simulink model "MultiMobileRobotObstacleAvoidance"  (R2020b)
settings: Solver=VariableStepAuto  StartTime=0.0  StopTime=100  RelTol=1e-3
values from neighbouring files (symbols this model uses):
  initTheta1 = -pi/2    (= -1.57079632679)    [createEnvMulti.m]
  initTheta2 = -pi/2    (= -1.57079632679)    [createEnvMulti.m]
  initX1 = 5    [createEnvMulti.m]
  initX2 = 22    [createEnvMulti.m]
  initY1 = 22    [createEnvMulti.m]
  initY2 = 22    [createEnvMulti.m]
  lidarNoiseSeeds = randi(intmax,size(scanAngles))    [createEnvMulti.m]
  lidarNoiseVariance = 0.1^2    (= 0.01)    [createEnvMulti.m]
  mapMatrix = simpleMap    [createEnvMulti.m]
  maxAngSpeed = 0.3    [createEnvMulti.m]
  maxLinSpeed = 0.3    [createEnvMulti.m]
  maxRange = 12    [createEnvMulti.m]
  sampleTime = 0.1    [createEnvMulti.m]
libraries: simulink x6, rllib x2, robotmobilelib x2
settings Model: Creator=fan  LastModifiedBy=fanyang

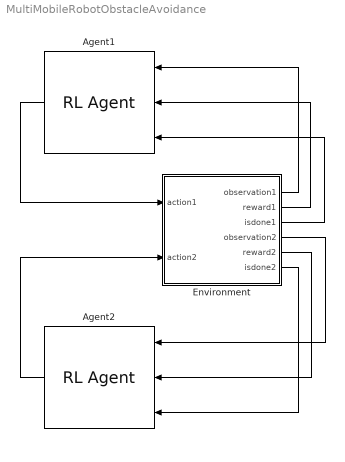
== system MultiMobileRobotObstacleAvoidance ==
  Agent1 : rllib/RL Agent  Agent=obstacleAvoidanceAgent1  ProvideReward=on  ProvideIsDone=on  ProvideCumRwd=off  TreatAsDirectFeedthrough=on  CollectLoggedSignals=on  CollectModelStates=on
  Agent2 : rllib/RL Agent  Agent=obstacleAvoidanceAgent2  ProvideReward=on  ProvideIsDone=on  ProvideCumRwd=off  TreatAsDirectFeedthrough=on  CollectLoggedSignals=on  CollectModelStates=on
  Environment : Subsystem
  wires:
  Environment/6(isdone2) -> Agent2/3
  Agent2/1 -> Environment/2(action2)
  Environment/3(isdone1) -> Agent1/3
  Environment/4(observation2) -> Agent2/1
  Environment/5(reward2) -> Agent2/2
  Environment/1(observation1) -> Agent1/1
  Environment/2(reward1) -> Agent1/2
  Agent1/1 -> Environment/1(action1)

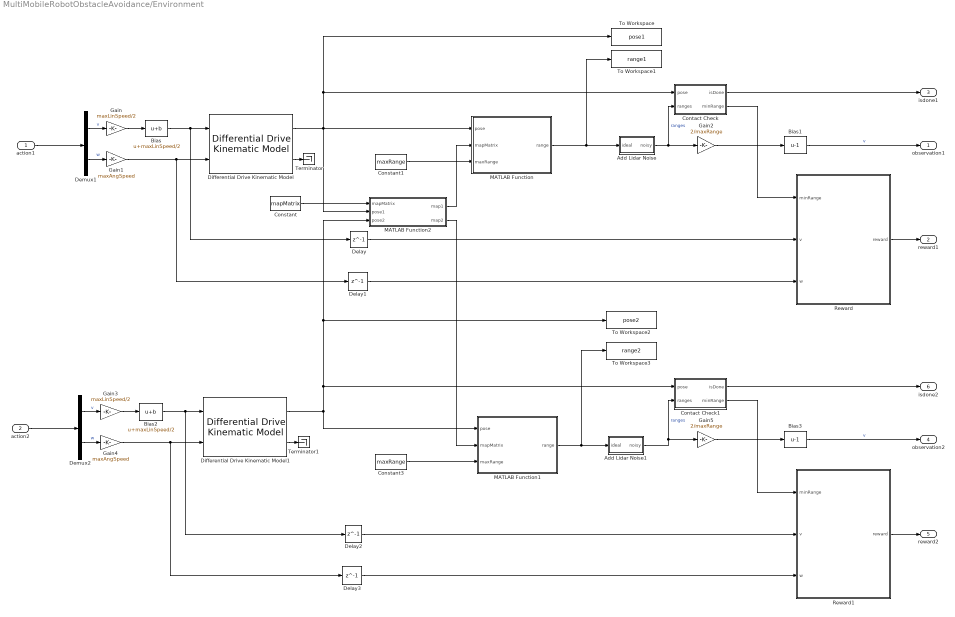
== system MultiMobileRobotObstacleAvoidance/Environment ==
  action1 : Inport
  action2 : Inport  Port=2
  Add Lidar Noise : Subsystem
  Add Lidar Noise1 : Subsystem
  Bias : Bias  Bias=maxLinSpeed/2
  Bias1 : Bias  Bias=-1
  Bias2 : Bias  Bias=maxLinSpeed/2
  Bias3 : Bias  Bias=-1
  Constant : Constant  Value=mapMatrix
  Constant1 : Constant  Value=maxRange
  Constant3 : Constant  Value=maxRange
  Contact Check : Subsystem
  Contact Check1 : Subsystem
  Delay{,1..3} (4 alike) : Delay  DelayLength=1  InitialCondition=0  UseCircularBuffer=on
  Demux1 : Demux  Outputs=2
  Demux2 : Demux  Outputs=2
  Differential Drive Kinematic Model : robotmobilelib/Differential Drive Kinematic Model  VehicleInputs=Vehicle Speed & Heading Angular Velocity  WheelRadius=0.05  WheelSpeedRange=[-inf inf]  TrackWidth=0.2  InitialState=[initX1; initY1; initTheta1]  SimulateUsing=Code generation
      settings: SourceProductBaseCode=RO
  Differential Drive Kinematic Model1 : robotmobilelib/Differential Drive Kinematic Model  VehicleInputs=Vehicle Speed & Heading Angular Velocity  WheelRadius=0.05  WheelSpeedRange=[-inf inf]  TrackWidth=0.2  InitialState=[initX2; initY2; initTheta2]  SimulateUsing=Code generation
      settings: SourceProductBaseCode=RO
  Gain : Gain  Gain=maxLinSpeed/2
  Gain1 : Gain  Gain=maxAngSpeed
  Gain2 : Gain  Gain=2/maxRange
  Gain3 : Gain  Gain=maxLinSpeed/2
  Gain4 : Gain  Gain=maxAngSpeed
  Gain5 : Gain  Gain=2/maxRange
  MATLAB Function : MATLAB Function  TreatAsAtomicUnit=on
  MATLAB Function1 : MATLAB Function  TreatAsAtomicUnit=on
  MATLAB Function2 : MATLAB Function  TreatAsAtomicUnit=on
  Reward : Subsystem
  Reward1 : Subsystem
  Terminator : Terminator
  Terminator1 : Terminator
  To Workspace : ToWorkspace  VariableName=pose1  SampleTime=-1
      settings: Save2DSignal=2-D array (concatenate along first dimension)
  To Workspace1 : ToWorkspace  VariableName=range1  SampleTime=-1
  To Workspace2 : ToWorkspace  VariableName=pose2  SampleTime=-1
      settings: Save2DSignal=2-D array (concatenate along first dimension)
  To Workspace3 : ToWorkspace  VariableName=range2  SampleTime=-1
  observation1 : Outport
  reward1 : Outport  Port=2
  isdone1 : Outport  Port=3
  observation2 : Outport  Port=4
  reward2 : Outport  Port=5
  isdone2 : Outport  Port=6
  wires:
  Differential Drive Kinematic Model/2 -> Terminator/1
  Differential Drive Kinematic Model/1 -> To Workspace/1, Contact Check/1(pose), MATLAB Function2/2(pose1), MATLAB Function/1(pose)
  action1/1 -> Demux1/1
  Bias/1 -> Delay/1, Differential Drive Kinematic Model/1
  Gain1/1 -> Delay1/1, Differential Drive Kinematic Model/2
  MATLAB Function/1(range) -> Add Lidar Noise/1(ideal), To Workspace1/1
  Contact Check/1(isDone) -> isdone1/1
  Contact Check/2(minRange) -> Reward/1(minRange)
  Reward/1(reward) -> reward1/1
  Gain2/1 -> Bias1/1
  Bias1/1 -> observation1/1  "v"
  Constant1/1 -> MATLAB Function/3(maxRange)
  Delay/1 -> Reward/2(v)
  Delay1/1 -> Reward/3(w)
  Demux1/2 -> Gain1/1  "w"
  Gain/1 -> Bias/1
  Demux1/1 -> Gain/1  "v"
  Add Lidar Noise/1(noisy) -> Gain2/1, Contact Check/2(ranges)  "ranges"
  Constant3/1 -> MATLAB Function1/3(maxRange)
  Delay2/1 -> Reward1/2(v)
  Add Lidar Noise1/1(noisy) -> Gain5/1, Contact Check1/2(ranges)  "ranges"
  Bias2/1 -> Delay2/1, Differential Drive Kinematic Model1/1
  Delay3/1 -> Reward1/3(w)
  Demux2/1 -> Gain3/1  "v"
  Demux2/2 -> Gain4/1  "w"
  Differential Drive Kinematic Model1/2 -> Terminator1/1
  Gain5/1 -> Bias3/1
  Gain3/1 -> Bias2/1
  action2/1 -> Demux2/1
  Reward1/1(reward) -> reward2/1
  Gain4/1 -> Delay3/1, Differential Drive Kinematic Model1/2
  Bias3/1 -> observation2/1  "v"
  Contact Check1/1(isDone) -> isdone2/1
  Contact Check1/2(minRange) -> Reward1/1(minRange)
  MATLAB Function1/1(range) -> To Workspace3/1, Add Lidar Noise1/1(ideal)
  Differential Drive Kinematic Model1/1 -> MATLAB Function2/3(pose2), To Workspace2/1, Contact Check1/1(pose), MATLAB Function1/1(pose)
  Constant/1 -> MATLAB Function2/1(mapMatrix)
  MATLAB Function2/1(map1) -> MATLAB Function/2(mapMatrix)
  MATLAB Function2/2(map2) -> MATLAB Function1/2(mapMatrix)

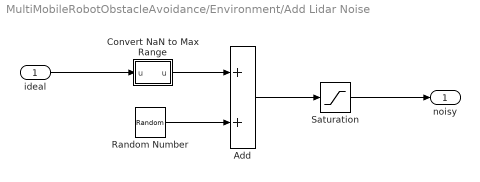
== system MultiMobileRobotObstacleAvoidance/Environment/Add Lidar Noise ==
  ideal : Inport
  Add : Sum
  Convert NaN to Max Range : MATLAB Function  TreatAsAtomicUnit=on
  Random Number : RandomNumber  Variance=lidarNoiseVariance  Seed=lidarNoiseSeeds  SampleTime=sampleTime
  Saturation : Saturate  UpperLimit=inf  LowerLimit=0
  noisy : Outport
  wires:
  Random Number/1 -> Add/2
  Add/1 -> Saturation/1
  Saturation/1 -> noisy/1
  ideal/1 -> Convert NaN to Max Range/1("u ")
  Convert NaN to Max Range/1(u) -> Add/1

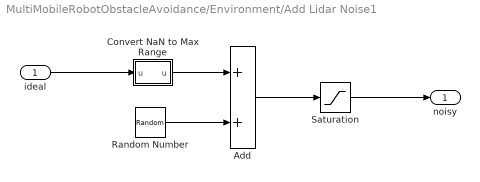
== system MultiMobileRobotObstacleAvoidance/Environment/Add Lidar Noise1 ==
  ideal : Inport
  Add : Sum
  Convert NaN to Max Range : MATLAB Function  TreatAsAtomicUnit=on
  Random Number : RandomNumber  Variance=lidarNoiseVariance  Seed=lidarNoiseSeeds  SampleTime=sampleTime
  Saturation : Saturate  UpperLimit=inf  LowerLimit=0
  noisy : Outport
  wires:
  Random Number/1 -> Add/2
  Add/1 -> Saturation/1
  Saturation/1 -> noisy/1
  ideal/1 -> Convert NaN to Max Range/1("u ")
  Convert NaN to Max Range/1(u) -> Add/1

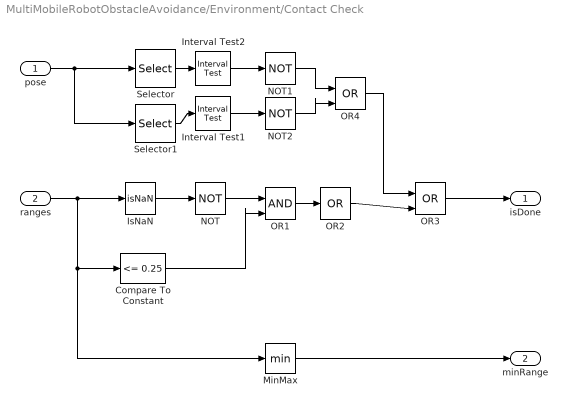
== system MultiMobileRobotObstacleAvoidance/Environment/Contact Check ==
  pose : Inport
  ranges : Inport  Port=2
  Compare To Constant : simulink/Logic and Bit Operations/Compare To Constant  relop=<=  const=0.25  OutDataTypeStr=boolean
  Interval Test1 : simulink/Logic and Bit Operations/Interval Test  IntervalClosedRight=on  uplimit=size(mapMatrix, 1)  IntervalClosedLeft=on  lowlimit=0  OutDataTypeStr=boolean
  Interval Test2 : simulink/Logic and Bit Operations/Interval Test  IntervalClosedRight=on  uplimit=size(mapMatrix, 2)  IntervalClosedLeft=on  lowlimit=0  OutDataTypeStr=boolean
  IsNaN : RelationalOperator  Operator=isNaN  OutDataTypeStr=boolean  RndMeth=Simplest
  MinMax : MinMax
  NOT : Logic  Operator=NOT  IconShape=distinctive  AllPortsSameDT=off  OutDataTypeStr=boolean
  NOT1 : Logic  Operator=NOT  IconShape=distinctive  AllPortsSameDT=off  OutDataTypeStr=boolean
  NOT2 : Logic  Operator=NOT  IconShape=distinctive  AllPortsSameDT=off  OutDataTypeStr=boolean
  OR1 : Logic  IconShape=distinctive  AllPortsSameDT=off  OutDataTypeStr=boolean
  OR2 : Logic  Operator=OR  Inputs=1  IconShape=distinctive  AllPortsSameDT=off  OutDataTypeStr=boolean
  OR3 : Logic  Operator=OR  IconShape=distinctive  AllPortsSameDT=off  OutDataTypeStr=boolean
  OR4 : Logic  Operator=OR  IconShape=distinctive  AllPortsSameDT=off  OutDataTypeStr=boolean
  Selector : Selector  InputPortWidth=3  IndexOptions=Index vector (dialog)  Indices=1  OutputSizes=1
  Selector1 : Selector  InputPortWidth=3  IndexOptions=Index vector (dialog)  Indices=2  OutputSizes=1
  isDone : Outport  VectorParamsAs1DForOutWhenUnconnected=off
  minRange : Outport  Port=2  VectorParamsAs1DForOutWhenUnconnected=off
  wires:
  OR1/1 -> OR2/1
  Compare To Constant/1 -> OR1/2
  NOT/1 -> OR1/1
  ranges/1 -> MinMax/1, Compare To Constant/1, IsNaN/1
  IsNaN/1 -> NOT/1
  MinMax/1 -> minRange/1
  OR3/1 -> isDone/1
  pose/1 -> Selector/1, Selector1/1
  Selector/1 -> Interval Test2/1
  Selector1/1 -> Interval Test1/1
  OR2/1 -> OR3/2
  NOT1/1 -> OR4/1
  Interval Test1/1 -> NOT2/1
  OR4/1 -> OR3/1
  Interval Test2/1 -> NOT1/1
  NOT2/1 -> OR4/2

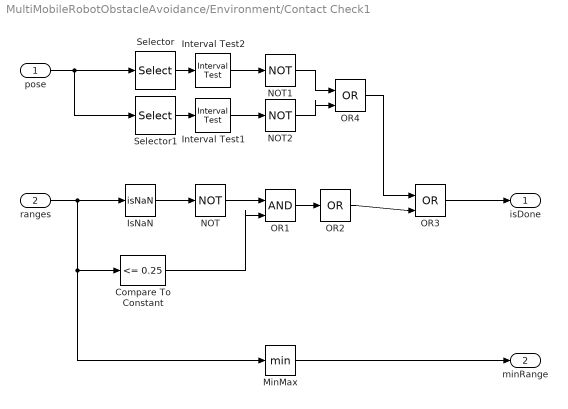
== system MultiMobileRobotObstacleAvoidance/Environment/Contact Check1 ==
  pose : Inport
  ranges : Inport  Port=2
  Compare To Constant : simulink/Logic and Bit Operations/Compare To Constant  relop=<=  const=0.25  OutDataTypeStr=boolean
  Interval Test1 : simulink/Logic and Bit Operations/Interval Test  IntervalClosedRight=on  uplimit=size(mapMatrix, 1)  IntervalClosedLeft=on  lowlimit=0  OutDataTypeStr=boolean
  Interval Test2 : simulink/Logic and Bit Operations/Interval Test  IntervalClosedRight=on  uplimit=size(mapMatrix, 2)  IntervalClosedLeft=on  lowlimit=0  OutDataTypeStr=boolean
  IsNaN : RelationalOperator  Operator=isNaN  OutDataTypeStr=boolean  RndMeth=Simplest
  MinMax : MinMax
  NOT : Logic  Operator=NOT  IconShape=distinctive  AllPortsSameDT=off  OutDataTypeStr=boolean
  NOT1 : Logic  Operator=NOT  IconShape=distinctive  AllPortsSameDT=off  OutDataTypeStr=boolean
  NOT2 : Logic  Operator=NOT  IconShape=distinctive  AllPortsSameDT=off  OutDataTypeStr=boolean
  OR1 : Logic  IconShape=distinctive  AllPortsSameDT=off  OutDataTypeStr=boolean
  OR2 : Logic  Operator=OR  Inputs=1  IconShape=distinctive  AllPortsSameDT=off  OutDataTypeStr=boolean
  OR3 : Logic  Operator=OR  IconShape=distinctive  AllPortsSameDT=off  OutDataTypeStr=boolean
  OR4 : Logic  Operator=OR  IconShape=distinctive  AllPortsSameDT=off  OutDataTypeStr=boolean
  Selector : Selector  InputPortWidth=3  IndexOptions=Index vector (dialog)  Indices=1  OutputSizes=1
  Selector1 : Selector  InputPortWidth=3  IndexOptions=Index vector (dialog)  Indices=2  OutputSizes=1
  isDone : Outport  VectorParamsAs1DForOutWhenUnconnected=off
  minRange : Outport  Port=2  VectorParamsAs1DForOutWhenUnconnected=off
  wires:
  OR1/1 -> OR2/1
  Compare To Constant/1 -> OR1/2
  NOT/1 -> OR1/1
  ranges/1 -> MinMax/1, Compare To Constant/1, IsNaN/1
  IsNaN/1 -> NOT/1
  MinMax/1 -> minRange/1
  OR3/1 -> isDone/1
  pose/1 -> Selector/1, Selector1/1
  Selector/1 -> Interval Test2/1
  Selector1/1 -> Interval Test1/1
  OR2/1 -> OR3/2
  NOT1/1 -> OR4/1
  Interval Test1/1 -> NOT2/1
  OR4/1 -> OR3/1
  Interval Test2/1 -> NOT1/1
  NOT2/1 -> OR4/2

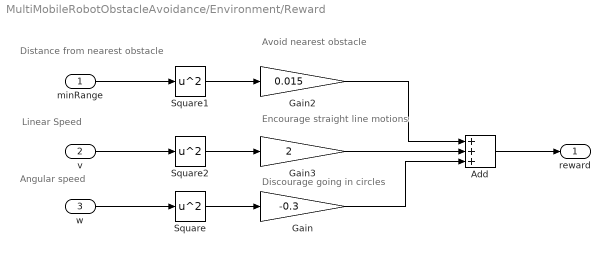
== system MultiMobileRobotObstacleAvoidance/Environment/Reward ==
  note: Discourage going in circles
  note: Encourage straight line motions
  note: Angular speed
  note: Linear Speed
  note: Distance from nearest obstacle
  note: Avoid nearest obstacle
  minRange : Inport
  v : Inport  Port=2
  w : Inport  Port=3
  Add : Sum  Inputs=+++
  Gain : Gain  Gain=-0.3
  Gain2 : Gain  Gain=0.015
  Gain3 : Gain  Gain=2
  Square : Math  Operator=square  SignedPower=on  SaturateOnIntegerOverflow=on
  Square1 : Math  Operator=square  SignedPower=on  SaturateOnIntegerOverflow=on
  Square2 : Math  Operator=square  SignedPower=on  SaturateOnIntegerOverflow=on
  reward : Outport  VectorParamsAs1DForOutWhenUnconnected=off
  wires:
  Square/1 -> Gain/1
  w/1 -> Square/1
  Gain/1 -> Add/3
  minRange/1 -> Square1/1
  Gain2/1 -> Add/1
  Square1/1 -> Gain2/1
  v/1 -> Square2/1
  Square2/1 -> Gain3/1
  Gain3/1 -> Add/2
  Add/1 -> reward/1

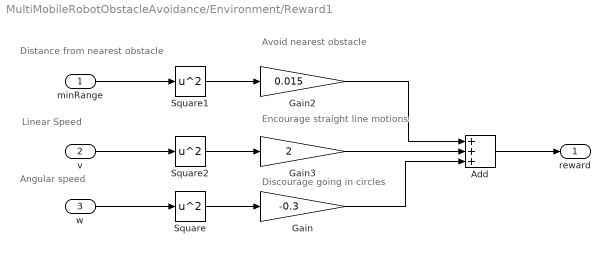
== system MultiMobileRobotObstacleAvoidance/Environment/Reward1 ==
  note: Discourage going in circles
  note: Encourage straight line motions
  note: Angular speed
  note: Linear Speed
  note: Distance from nearest obstacle
  note: Avoid nearest obstacle
  minRange : Inport
  v : Inport  Port=2
  w : Inport  Port=3
  Add : Sum  Inputs=+++
  Gain : Gain  Gain=-0.3
  Gain2 : Gain  Gain=0.015
  Gain3 : Gain  Gain=2
  Square : Math  Operator=square  SignedPower=on  SaturateOnIntegerOverflow=on
  Square1 : Math  Operator=square  SignedPower=on  SaturateOnIntegerOverflow=on
  Square2 : Math  Operator=square  SignedPower=on  SaturateOnIntegerOverflow=on
  reward : Outport  VectorParamsAs1DForOutWhenUnconnected=off
  wires:
  Square/1 -> Gain/1
  w/1 -> Square/1
  Gain/1 -> Add/3
  minRange/1 -> Square1/1
  Gain2/1 -> Add/1
  Square1/1 -> Gain2/1
  v/1 -> Square2/1
  Square2/1 -> Gain3/1
  Gain3/1 -> Add/2
  Add/1 -> reward/1

== matlab function MultiMobileRobotObstacleAvoidance/Environment/MATLAB Function ==
  settings: updateMethod=DISCRETE
  data: range output size=[7, 1]; pose input size=[3, 1]; mapMatrix input size=[size(mapMatrix, 1), size(mapMatrix, 2)]; maxRange input; mapScale parameter
function range = RangeSensor(pose, mapMatrix, maxRange, mapScale)
persistent r
if isempty(r)
 r = rangeSensor('HorizontalAngle', [-3*pi/8, 3*pi/8], 'HorizontalAngleResolution', pi/8, 'Range', [0 maxRange]);
end
range = r(pose', binaryOccupancyMap(mapMatrix, mapScale));
end

== matlab function MultiMobileRobotObstacleAvoidance/Environment/Add Lidar Noise/Convert NaN to Max Range ==
  data: u input; u output; maxRange parameter
function u = removeNans(u,maxRange)

u(isnan(u)) = maxRange;

== matlab function MultiMobileRobotObstacleAvoidance/Environment/Add Lidar Noise1/Convert NaN to Max Range ==
  data: u input; u output; maxRange parameter
function u = removeNans(u,maxRange)

u(isnan(u)) = maxRange;

== matlab function MultiMobileRobotObstacleAvoidance/Environment/MATLAB Function1 ==
  settings: updateMethod=DISCRETE
  data: range output size=[7, 1]; pose input size=[3, 1]; mapMatrix input size=[size(mapMatrix, 1), size(mapMatrix, 2)]; maxRange input; mapScale parameter
function range = RangeSensor(pose, mapMatrix, maxRange, mapScale)
persistent r
if isempty(r)
 r = rangeSensor('HorizontalAngle', [-3*pi/8, 3*pi/8], 'HorizontalAngleResolution', pi/8, 'Range', [0 maxRange]);
end
range = r(pose', binaryOccupancyMap(mapMatrix, mapScale));
end

== matlab function MultiMobileRobotObstacleAvoidance/Environment/MATLAB Function2 ==
  data: mapMatrix input; map1 output; pose1 input; map2 output; pose2 input
function [map1, map2] = updateMap(mapMatrix, pose1, pose2)
mmp = binaryOccupancyMap(mapMatrix);
[xlim, ylim] = size(mapMatrix);
% poses = [pose1; pose2];
% poses_grid = world2grid(mmp, [poses(:,1),poses(:,2)]);
poses_grid1 = world2grid(mmp, [pose2(1),pose2(2)]);
map1 = mapMatrix;
if poses_grid1(1) > 0 && poses_grid1(2) > 0 && poses_grid1(1) <= xlim && poses_grid1(2) <= ylim
    map1(poses_grid1(1), poses_grid1(2)) = true;
end

poses_grid2 = world2grid(mmp, [pose1(1),pose1(2)]);
map2 = mapMatrix;
if poses_grid2(1) > 0 && poses_grid2(2) > 0 && poses_grid2(1) <= xlim && poses_grid2(2) <= ylim
    map2(poses_grid2(1), poses_grid2(2)) = true; 
end
